simulink model "BuckBoost"  (R2018b)
settings: Solver=FixedStepDiscrete  StartTime=0.0  StopTime=10.0  RelTol=1e-3  EnableMultiTasking=on
libraries: HRTIMERS_Lib x12, GPIO_Lib x3, ADC_Lib x1, STM32_Config_Lib x1
settings Model: Creator=reynaudp  LastModifiedBy=fenard1
settings DataIOCC: LimitDataPoints=on  SaveFormat=Array
settings OptimizationCC: DefaultParameterBehavior=Inlined  LifeSpan=1
settings DebuggingCC: SolverPrmCheckMsg=warning  MultiTaskDSMMsg=none  AllowSymbolicDim=off  SFUnexpectedBacktrackingDiag=warning  SFNoUnconditionalDefaultTransitionDiag=warning  SFExecutionAtInitializationDiag=none
settings HardwareCC: ProdBitPerPointer=32  ProdBitPerSizeT=32  ProdBitPerPtrDiffT=32  ProdLargestAtomicInteger=Integer  ProdWordSize=32  ProdHWDeviceType=STMicroelectronics->STM32 32-bit Cortex-M
settings ModelReferenceCC: PropagateSignalLabelsOutOfModel=off
settings SFSimCC: SimUseLocalCustomCode=off  MATLABDynamicMemAlloc=off
settings RTWCC: SystemTargetFile=stm32.tlc  TemplateMakefile=stm32.tmf  Description=stm32 (Embedded Target)  GenerateReport=on  RTWUseLocalCustomCode=off
settings CodeAppCC: IgnoreCustomStorageClasses=off  CustomSymbolStrType=$N$R$M  SimulinkBlockComments=off
settings STFCustomTargetCC: CodeReplacementLibrary=ARM CMSIS SIN COS  ParMdlRefBuildCompliant=on  IncludeMdlTerminateFcn=off  CombineOutputUpdateFcns=on  ERTCustomFileBanners=on  SupportNonFinite=off  SupportComplex=off  SupportContinuousTime=off  SupportNonInlinedSFcns=off  RemoveResetFunc=on  MATLABClassNameForMDSCustomization=Simulink.SoftwareTarget.ERTCustomization  SystemTargetFile=stm32.tlc
settings ERTTargetCC: CodeReplacementLibrary=ARM CMSIS SIN COS  MultiwordLength=2048  CompOptLevelCompliant=off  ConcurrentExecutionCompliant=off  IncludeMdlTerminateFcn=off  SupportNonFinite=off  SupportComplex=off  ModelStepFunctionPrototypeControlCompliant=off  CPPClassGenCompliant=off  UseToolchainInfoCompliant=off  ERTSrcFileBannerTemplate=sourceFileTemplate.cgt  ERTHdrFileBannerTemplate=sourceFileTemplate.cgt  ERTDataSrcFileTemplate=sourceFileTemplate.cgt  ERTDataHdrFileTemplate=sourceFileTemplate.cgt  ERTCustomFileTemplate=customRoutineProcess.tlc  ConvertIfToSwitch=off  SuppressUnreachableDefaultCases=off
settings ConfigComp: CovMetricSettings=dw  CovHtmlReporting=on  CovSaveCumulativeToWorkspaceVar=on  CovSaveSingleToWorkspaceVar=on  CovExternalEMLEnable=off  CovSFcnEnable=off

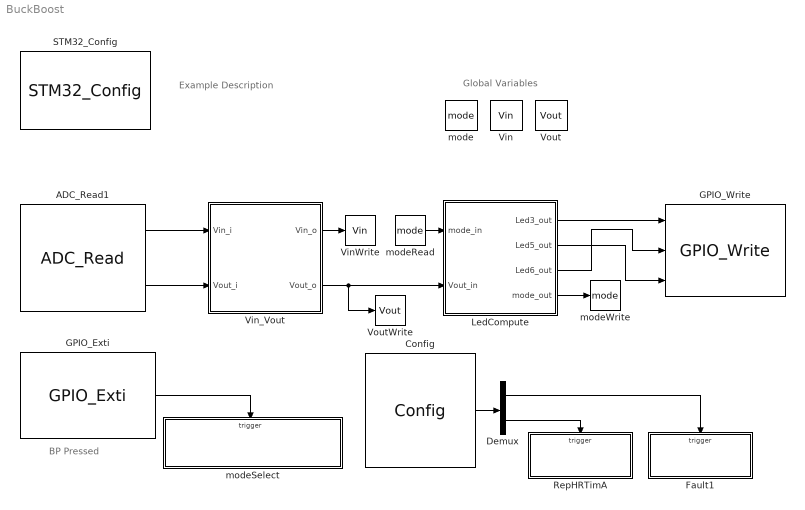
== system BuckBoost ==
  note: Example Description
  note: Global Variables
  note: BP Pressed
  ADC_Read1 : ADC_Lib/ADC_Read  ADC_Name=ADC1  ADC_Ch0=off  ADC_Ch1=off  ADC_Ch2=on  ADC_Ch3=off  ADC_Ch4=on  ADC_Ch5=off  ADC_Ch6=off  ADC_Ch7=off  ADC_Ch8=off  ADC_Ch9=off  ADC_Ch10=off  ADC_Ch11=off  ADC_Ch12=off  ADC_Ch13=off  ADC_Ch14=off  ADC_Ch15=off  ADC_Ch16=off  ADC_Ch17=off  ADC_Ch18=off  RgRk1=off  RgRk2=off  RgRk3=off  RgRk4=off  RgRk1_Ch=off  RgRk2_Ch=off  RgRk3_Ch=off  RgRk4_Ch=off  RgRk5=off  RgRk6=off  RgRk7=off  RgRk8=off  RgRk5_Ch=off  RgRk6_Ch=off  RgRk7_Ch=off  RgRk8_Ch=off  RgRk9=off  RgRk10=off  RgRk11=off  RgRk12=off  RgRk9_Ch=off  RgRk10_Ch=off  RgRk11_Ch=off  RgRk12_Ch=off  RgRk13=off  RgRk14=off  RgRk15=off  RgRk16=off  RgRk13_Ch=off  RgRk14_Ch=off  RgRk15_Ch=off  RgRk16_Ch=off  InjRk1=on  InjRk2=on  InjRk3=off  InjRk4=off  InjRk1_Ch=Ch2_i1  InjRk2_Ch=Ch4_i2  InjRk3_Ch=off  InjRk4_Ch=off  ADC_Trig=Not used  ADC_TrigEdge=Not used  DmaReq=off  DMA_Buffer=0  ItReq=off  AWD_Mode=NOT_USED  AWD_Ch=0  AWD_HThres=0  AWD_LThres=0  AWD_En_Int=off  AWD2_HThres=0  AWD2_LThres=0  AWD2_En_Int=off  AWD3_HThres=0  AWD3_LThres=0  AWD3_En_Int=off  EOC_SEQ=off  EOC_IT=off  JEOC_IT=off  AWD_IT=off  OVR_IT=off  CpltTrans=off  HalfTrans=off  ADC_RegNb=0  ADC_RegCh0=off  ADC_RegCh1=off  ADC_RegCh2=off  ADC_RegCh3=off  ADC_RegCh4=off  ADC_RegCh5=off  ADC_RegCh6=off  ADC_RegCh7=off  ADC_RegCh8=off  ADC_RegCh9=off  ADC_RegCh10=off  ADC_RegCh11=off  ADC_RegCh12=off  ADC_RegCh13=off  ADC_RegCh14=off  ADC_RegCh15=off  ADC_RegCh16=off  ADC_RegCh17=off  ADC_RegCh18=off  ADC_InjNb=2  ADC_InjCh0=off  ADC_InjCh1=off  ADC_InjCh2=on  ADC_InjCh3=off  ADC_InjCh4=on  ADC_InjCh5=off  ADC_InjCh6=off  ADC_InjCh7=off  ADC_InjCh8=off  ADC_InjCh9=off  ADC_InjCh10=off  ADC_InjCh11=off  ADC_InjCh12=off  ADC_InjCh13=off  ADC_InjCh14=off  ADC_InjCh15=off  ADC_InjCh16=off  ADC_InjCh17=off  ADC_InjCh18=off  ADC_RegRank0=0  ADC_RegRank1=0  ADC_RegRank2=0  ADC_RegRank3=0  ADC_RegRank4=0  ADC_RegRank5=0  ADC_RegRank6=0  ADC_RegRank7=0  ADC_RegRank8=0  ADC_RegRank9=0  ADC_RegRank10=0  ADC_RegRank11=0  ADC_RegRank12=0  ADC_RegRank13=0  ADC_RegRank14=0  ADC_RegRank15=0  ADC_RegRank16=0  ADC_RegRank17=0  ADC_RegRank18=0  ADC_InjRank0=0  ADC_InjRank1=0  ADC_InjRank2=1  ADC_InjRank3=0  ADC_InjRank4=2  ADC_InjRank5=0  ADC_InjRank6=0  ADC_InjRank7=0  ADC_InjRank8=0  ADC_InjRank9=0  ADC_InjRank10=0  ADC_InjRank11=0  ADC_InjRank12=0  ADC_InjRank13=0  ADC_InjRank14=0  ADC_InjRank15=0  ADC_InjRank16=0  ADC_InjRank17=0  ADC_InjRank18=0  NbADC=1  CurrentADC=ADC1
      settings: SourceProductName=Target Support Package - STM32 Adapter
  Config : HRTIMERS_Lib/Config  currentHRTIM=HRTIM1  NbHRTim=1  HRTIM_Name=HRTIM1  HRTIM_Clock=144000000  TIM_IRQ_F1=on  TIM_IRQ_F2=off  TIM_IRQ_F3=off  TIM_IRQ_F4=off  TIM_IRQ_F5=off  TIM_IRQ_F6=off  TIM_IRQ_SF=off  TIM_IRQ_BMP=off  TIM_IRQ_DLLCALL=off  TIM_IRQ_SYNC=off  TIM_IRQ_BURST_DMA=off  TIM_IRQ_DMA_ERR=off  M_DMA=off  M_IT_global=off  M_Tim_div=MUL32  M_Period=0  M_PWM_Period=Inf  M_Unit1=0  M_Unit2=0  M_Unit3=0  M_Unit4=0  TIM_IRQ_UPDM=off  TIM_IRQ_REPM=off  TIM_IRQ_COMP1=off  TIM_IRQ_COMP2=off  TIM_IRQ_COMP3=off  TIM_IRQ_COMP4=off  A_Mode=Advanced  A_DMA=off  A_IT_global=on  A_Tim_div=MUL32  A_Period=18432  A_PWM_Period=250000  A_Capture1=off  A_Capture2=off  TA1_Enable=on  TA1_Polarity=HIGH  TA1_Chopper=off  TA2_Enable=on  TA2_Polarity=HIGH  TA2_Chopper=off  A_Unit1=18336  A_Unit2=9216  A_Unit3=0  A_Unit4=0  A_Output_Comp1=off  A_Comp_Polarity1=HIGH  A_CompVal1=0  A_Output_Comp2=off  A_Comp_Polarity2=HIGH  A_CompVal2=0  A_Output_PWM1=off  A_Output_Polarity1=HIGH  A_DutyVal1=0  A_DutyIn1=off  A_Output_PWM2=off  A_Output_Polarity2=HIGH  A_DutyVal2=0  A_DutyIn2=off  A_OnePulse1=off  A_OnePulse_Polarity1=HIGH  A_OnePulse_CompVal1=0  A_OnePulse2=off  A_OnePulse_Polarity2=HIGH  A_OnePulse_CompVal2=0  TIM_IRQ_UPDA=off  TIM_IRQ_REPA=on  TIM_IRQ_COMP1A=off  TIM_IRQ_COMP2A=off  TIM_IRQ_COMP3A=off  TIM_IRQ_COMP4A=off  TIM_IRQ_CAPT1A=off  TIM_IRQ_CAPT2A=off  TIM_IRQ_DELA=off  TIM_IRQ_RESET_CPTA=off  TIM_IRQ_OUT1SA=off  TIM_IRQ_OUT1RA=off  TIM_IRQ_OUT2SA=off  TIM_IRQ_OUT2RA=off  B_Mode=Advanced  B_DMA=off  B_IT_global=off  B_Tim_div=MUL32  B_Period=18432  B_PWM_Period=250000  B_Capture1=off  B_Capture2=off  TB1_Enable=on  TB1_Polarity=HIGH  TB1_Chopper=off  TB2_Enable=on  TB2_Polarity=HIGH  TB2_Chopper=off  B_Unit1=18433  B_Unit2=0  B_Unit3=0  B_Unit4=0  B_Output_Comp1=off  B_Comp_Polarity1=HIGH  B_CompVal1=0  B_Output_Comp2=off  B_Comp_Polarity2=HIGH  B_CompVal2=0  B_Output_PWM1=off  B_Output_Polarity1=HIGH  B_DutyVal1=0  B_DutyIn1=off  B_Output_PWM2=off  B_Output_Polarity2=HIGH  B_DutyVal2=0  B_DutyIn2=off  B_OnePulse1=off  B_OnePulse_Polarity1=HIGH  B_OnePulse_CompVal1=0  B_OnePulse2=off  B_OnePulse_Polarity2=HIGH  B_OnePulse_CompVal2=0  TIM_IRQ_UPDB=off  TIM_IRQ_REPB=off  TIM_IRQ_COMP1B=off  TIM_IRQ_COMP2B=off  TIM_IRQ_COMP3B=off  TIM_IRQ_COMP4B=off  TIM_IRQ_CAPT1B=off  TIM_IRQ_CAPT2B=off  TIM_IRQ_DELB=off  TIM_IRQ_RESET_CPTB=off  TIM_IRQ_OUT1SB=off  TIM_IRQ_OUT1RB=off  TIM_IRQ_OUT2SB=off  TIM_IRQ_OUT2RB=off  C_Mode=Advanced  C_DMA=off  C_IT_global=off  C_Tim_div=MUL32  C_Period=0  C_PWM_Period=Inf  C_Capture1=off  C_Capture2=off  TC1_Enable=off  TC1_Polarity=HIGH  TC1_Chopper=off  TC2_Enable=off  TC2_Polarity=HIGH  TC2_Chopper=off  C_Unit1=0  C_Unit2=0  C_Unit3=0  C_Unit4=0  C_Output_Comp1=off  C_Comp_Polarity1=HIGH  C_CompVal1=0  C_Output_Comp2=off  C_Comp_Polarity2=HIGH  C_CompVal2=0  C_Output_PWM1=off  C_Output_Polarity1=HIGH  C_DutyVal1=0  C_DutyIn1=off  C_Output_PWM2=off  C_Output_Polarity2=HIGH  C_DutyVal2=0  C_DutyIn2=off  C_OnePulse1=off  C_OnePulse_Polarity1=HIGH  C_OnePulse_CompVal1=0  C_OnePulse2=off  C_OnePulse_Polarity2=HIGH  C_OnePulse_CompVal2=0  TIM_IRQ_UPDC=off  TIM_IRQ_REPC=off  TIM_IRQ_COMP1C=off  TIM_IRQ_COMP2C=off  TIM_IRQ_COMP3C=off  TIM_IRQ_COMP4C=off  TIM_IRQ_CAPT1C=off  TIM_IRQ_CAPT2C=off  TIM_IRQ_DELC=off  TIM_IRQ_RESET_CPTC=off  TIM_IRQ_OUT1SC=off  TIM_IRQ_OUT1RC=off  TIM_IRQ_OUT2SC=off  TIM_IRQ_OUT2RC=off  D_Mode=Advanced  D_DMA=off  D_IT_global=off  D_Tim_div=MUL32  D_Period=0  D_PWM_Period=Inf  D_Capture1=off  D_Capture2=off  TD1_Enable=off  TD1_Polarity=HIGH  TD1_Chopper=off  TD2_Enable=off  TD2_Polarity=HIGH  TD2_Chopper=off  D_Unit1=0  D_Unit2=0  D_Unit3=0  D_Unit4=0  D_Output_Comp1=off  D_Comp_Polarity1=HIGH  D_CompVal1=0  D_Output_Comp2=off  D_Comp_Polarity2=HIGH  D_CompVal2=0  D_Output_PWM1=off  D_Output_Polarity1=HIGH  D_DutyVal1=0  D_DutyIn1=off  D_Output_PWM2=off  D_Output_Polarity2=HIGH  D_DutyVal2=0  D_DutyIn2=off  D_OnePulse1=off  D_OnePulse_Polarity1=HIGH  D_OnePulse_CompVal1=0  D_OnePulse2=off  D_OnePulse_Polarity2=HIGH  D_OnePulse_CompVal2=0  TIM_IRQ_UPDD=off  TIM_IRQ_REPD=off  TIM_IRQ_COMP1D=off  TIM_IRQ_COMP2D=off  TIM_IRQ_COMP3D=off  TIM_IRQ_COMP4D=off  TIM_IRQ_CAPT1D=off  TIM_IRQ_CAPT2D=off  TIM_IRQ_DELD=off  TIM_IRQ_RESET_CPTD=off  TIM_IRQ_OUT1SD=off  TIM_IRQ_OUT1RD=off  TIM_IRQ_OUT2SD=off  TIM_IRQ_OUT2RD=off  E_Mode=Advanced  E_DMA=off  E_IT_global=off  E_Tim_div=MUL32  E_Period=0  E_PWM_Period=Inf  E_Capture1=off  E_Capture2=off  TE1_Enable=off  TE1_Polarity=HIGH  TE1_Chopper=off  TE2_Enable=off  TE2_Polarity=HIGH  TE2_Chopper=off  E_Unit1=0  E_Unit2=0  E_Unit3=0  E_Unit4=0  E_Output_Comp1=off  E_Comp_Polarity1=HIGH  E_CompVal1=0  E_Output_Comp2=off  E_Comp_Polarity2=HIGH  E_CompVal2=0  E_Output_PWM1=off  E_Output_Polarity1=HIGH  E_DutyVal1=0  E_DutyIn1=off  E_Output_PWM2=off  E_Output_Polarity2=HIGH  E_DutyVal2=0  E_DutyIn2=off  E_OnePulse1=off  E_OnePulse_Polarity1=HIGH  E_OnePulse_CompVal1=0  E_OnePulse2=off  E_OnePulse_Polarity2=HIGH  E_OnePulse_CompVal2=0  TIM_IRQ_UPDE=off  TIM_IRQ_REPE=off  TIM_IRQ_COMP1E=off  TIM_IRQ_COMP2E=off  TIM_IRQ_COMP3E=off  TIM_IRQ_COMP4E=off  TIM_IRQ_CAPT1E=off  TIM_IRQ_CAPT2E=off  TIM_IRQ_DELE=off  TIM_IRQ_RESET_CPTE=off  TIM_IRQ_OUT1SE=off  TIM_IRQ_OUT1RE=off  TIM_IRQ_OUT2SE=off  TIM_IRQ_OUT2RE=off  F_Mode=Advanced  F_DMA=off  F_IT_global=off  F_Tim_div=MUL32  F_Period=0  F_PWM_Period=Inf  F_Capture1=off  F_Capture2=off  TF1_Enable=off  TF1_Polarity=HIGH  TF1_Chopper=off  TF2_Enable=off  TF2_Polarity=HIGH  TF2_Chopper=off  F_Unit1=0  F_Unit2=0  F_Unit3=0  F_Unit4=0  F_Output_Comp1=off  F_Comp_Polarity1=HIGH  F_CompVal1=0  F_Output_Comp2=off  F_Comp_Polarity2=HIGH  F_CompVal2=0  F_Output_PWM1=off  F_Output_Polarity1=HIGH  F_DutyVal1=0  F_DutyIn1=off  F_Output_PWM2=off  F_Output_Polarity2=HIGH  F_DutyVal2=0  F_DutyIn2=off  F_OnePulse1=off  F_OnePulse_Polarity1=HIGH  F_OnePulse_CompVal1=0  F_OnePulse2=off  F_OnePulse_Polarity2=HIGH  F_OnePulse_CompVal2=0  TIM_IRQ_UPDF=off  TIM_IRQ_REPF=off  TIM_IRQ_COMP1F=off  TIM_IRQ_COMP2F=off  TIM_IRQ_COMP3F=off  TIM_IRQ_COMP4F=off  TIM_IRQ_CAPT1F=off  TIM_IRQ_CAPT2F=off  TIM_IRQ_DELF=off  TIM_IRQ_RESET_CPTF=off  TIM_IRQ_OUT1SF=off  TIM_IRQ_OUT1RF=off  TIM_IRQ_OUT2SF=off  TIM_IRQ_OUT2RF=off  M_Used=off  A_Used=on  B_Used=on  C_Used=off  D_Used=off  E_Used=off  F_Used=off
      settings: SourceProductName=Target Support Package - STM32 Adapter
  Demux : Demux  Outputs=2
  Fault1 : Subsystem  TreatAsAtomicUnit=on
  GPIO_Exti : GPIO_Lib/GPIO_Exti  Priority=0  Port_name=GPIOA  Pin_0=on  Pin_1=off  Pin_2=off  Pin_3=off  Pin_4=off  Pin_5=off  Pin_6=off  Pin_7=off  Pin_8=off  Pin_9=off  Pin_10=off  Pin_11=off  Pin_12=off  Pin_13=off  Pin_14=off  Pin_15=off  PinList=GPIOA0
      settings: SourceProductName=Target Support Package - STM32 Adapter
  GPIO_Write : GPIO_Lib/GPIO_Write  Port_name=GPIOB  Pin0=off  Toggle_Pin0=off  Pin1=off  Toggle_Pin1=off  Pin2=off  Toggle_Pin2=off  Pin3=off  Toggle_Pin3=off  Pin4=off  Toggle_Pin4=off  Pin5=off  Toggle_Pin5=off  Pin6=on  Toggle_Pin6=off  Pin7=on  Toggle_Pin7=off  Pin8=off  Toggle_Pin8=off  Pin9=on  Toggle_Pin9=off  Pin10=off  Toggle_Pin10=off  Pin11=off  Toggle_Pin11=off  Pin12=off  Toggle_Pin12=off  Pin13=off  Toggle_Pin13=off  Pin14=off  Toggle_Pin14=off  Pin15=off  Toggle_Pin15=off  PinList="GPIOB6  7  8  9"
      settings: SourceProductName=Target Support Package - STM32 Adapter
  LedCompute : MATLAB Function  TreatAsAtomicUnit=on
  RepHRTimA : Subsystem  TreatAsAtomicUnit=on
  STM32_Config : STM32_Config_Lib/STM32_Config  Priority=0  Project_Path=.\  Config_File=BuckBoost.ioc  MCU_Name=STM32F334C8Tx
      settings: SourceProductName=Target Support Package - STM32 Adapter
  Vin : DataStoreMemory  DataStoreName=Vin  ReadBeforeWriteMsg=warning  WriteAfterWriteMsg=warning  WriteAfterReadMsg=warning  ShowAdditionalParam=off  OutMin=0  OutMax=5000  OutDataTypeStr=uint32
  VinWrite : DataStoreWrite  DataStoreName=Vin
  Vin_Vout : MATLAB Function  TreatAsAtomicUnit=on
  Vout : DataStoreMemory  DataStoreName=Vout  ReadBeforeWriteMsg=warning  WriteAfterWriteMsg=warning  WriteAfterReadMsg=warning  ShowAdditionalParam=off  OutMin=0  OutDataTypeStr=uint32
  VoutWrite : DataStoreWrite  DataStoreName=Vout
  mode : DataStoreMemory  DataStoreName=mode  ReadBeforeWriteMsg=warning  WriteAfterWriteMsg=warning  WriteAfterReadMsg=warning  ShowAdditionalParam=off  OutMin=0  OutMax=3  OutDataTypeStr=uint8
  modeRead : DataStoreRead  DataStoreName=mode
  modeSelect : Subsystem  TreatAsAtomicUnit=on
  modeWrite : DataStoreWrite  DataStoreName=mode
  wires:
  GPIO_Exti/1 -> modeSelect/Trigger
  ADC_Read1/2 -> Vin_Vout/2(Vout_i)
  ADC_Read1/1 -> Vin_Vout/1(Vin_i)
  Vin_Vout/1(Vin_o) -> VinWrite/1
  Vin_Vout/2(Vout_o) -> VoutWrite/1, LedCompute/2(Vout_in)
  modeRead/1 -> LedCompute/1(mode_in)
  LedCompute/4(mode_out) -> modeWrite/1
  LedCompute/1(Led3_out) -> GPIO_Write/1
  LedCompute/2(Led5_out) -> GPIO_Write/3
  LedCompute/3(Led6_out) -> GPIO_Write/2
  Config/1 -> Demux/1
  Demux/1 -> Fault1/Trigger
  Demux/2 -> RepHRTimA/Trigger

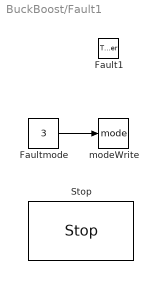
== system BuckBoost/Fault1 ==
  Fault1 : TriggerPort  TriggerType=function-call  VariantControl=Variant
  Faultmode : Constant  Value=3  OutDataTypeStr=uint8
  Stop : HRTIMERS_Lib/Stop  currentHRTIM=HRTIM1  NbHRTim=1  HRTIM_Name=HRTIM1  TA1_Stop=on  TA2_Stop=on  TB1_Stop=on  TB2_Stop=on  TC1_Stop=off  TC2_Stop=off  TD1_Stop=off  TD2_Stop=off  TE1_Stop=off  TE2_Stop=off  TF1_Stop=off  TF2_Stop=off
      settings: SourceProductName=Target Support Package - STM32 Adapter
  modeWrite : DataStoreWrite  DataStoreName=mode
  wires:
  Faultmode/1 -> modeWrite/1

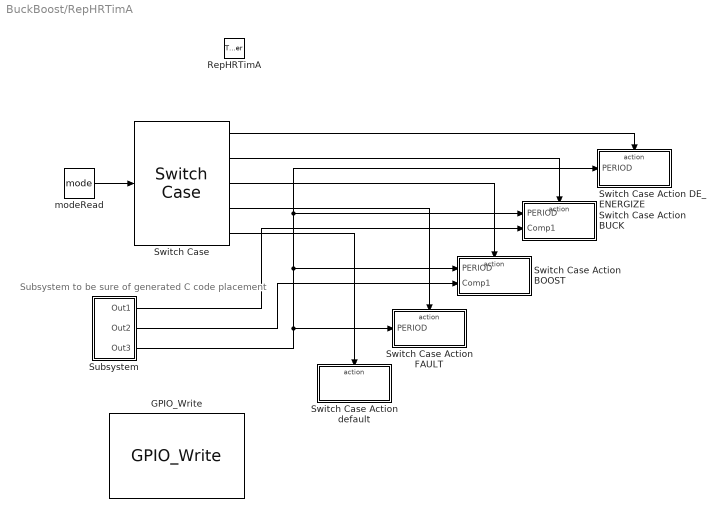
== system BuckBoost/RepHRTimA ==
  note: Subsystem to be sure of generated C code placement
  RepHRTimA : TriggerPort  TriggerType=function-call  VariantControl=Variant
  GPIO_Write : GPIO_Lib/GPIO_Write  Port_name=GPIOB  Pin0=off  Toggle_Pin0=off  Pin1=off  Toggle_Pin1=off  Pin2=off  Toggle_Pin2=off  Pin3=off  Toggle_Pin3=off  Pin4=off  Toggle_Pin4=off  Pin5=off  Toggle_Pin5=off  Pin6=off  Toggle_Pin6=off  Pin7=off  Toggle_Pin7=off  Pin8=on  Toggle_Pin8=on  Pin9=off  Toggle_Pin9=off  Pin10=off  Toggle_Pin10=off  Pin11=off  Toggle_Pin11=off  Pin12=off  Toggle_Pin12=off  Pin13=off  Toggle_Pin13=off  Pin14=off  Toggle_Pin14=off  Pin15=off  Toggle_Pin15=off  PinList="GPIOB6  7  8  9"
      settings: SourceProductName=Target Support Package - STM32 Adapter
  Subsystem : Subsystem  TreatAsAtomicUnit=on
      settings: RTWSystemCode=Inline
  Switch Case : SwitchCase  Priority=0  CaseConditions={0,1,2,3}
  Switch Case Action BOOST : Subsystem  TreatAsAtomicUnit=on
  Switch Case Action BUCK : Subsystem  TreatAsAtomicUnit=on
  Switch Case Action DE_ENERGIZE : Subsystem  TreatAsAtomicUnit=on
  Switch Case Action FAULT : Subsystem  TreatAsAtomicUnit=on
  Switch Case Action default : Subsystem  TreatAsAtomicUnit=on
  modeRead : DataStoreRead  DataStoreName=mode
  wires:
  modeRead/1 -> Switch Case/1
  Switch Case/2 -> Switch Case Action BUCK/Action
  Switch Case/3 -> Switch Case Action BOOST/Action
  Switch Case/4 -> Switch Case Action FAULT/Action
  Switch Case/1 -> Switch Case Action DE_ENERGIZE/Action
  Switch Case/5 -> Switch Case Action default/Action
  Subsystem/3(Out3) -> Switch Case Action BOOST/1(PERIOD), Switch Case Action BUCK/1(PERIOD), Switch Case Action DE_ENERGIZE/1(PERIOD), Switch Case Action FAULT/1(PERIOD)
  Subsystem/1(Out1) -> Switch Case Action BUCK/2(Comp1)
  Subsystem/2(Out2) -> Switch Case Action BOOST/2(Comp1)

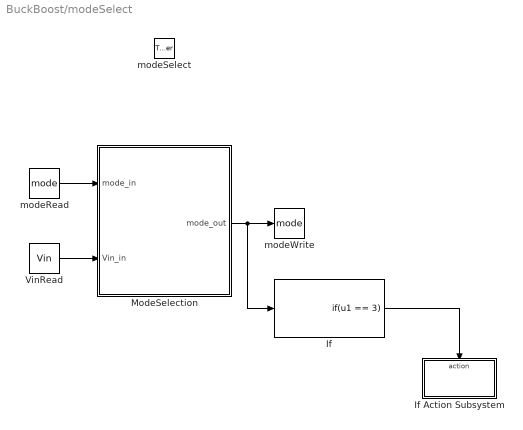
== system BuckBoost/modeSelect ==
  modeSelect : TriggerPort  TriggerType=function-call  VariantControl=Variant
  If : If  IfExpression=u1 == 3  ShowElse=off
  If Action Subsystem : Subsystem  TreatAsAtomicUnit=on
  ModeSelection : MATLAB Function  TreatAsAtomicUnit=on
  VinRead : DataStoreRead  DataStoreName=Vin
  modeRead : DataStoreRead  DialogController=Simulink.DDGSource  DataStoreName=mode
  modeWrite : DataStoreWrite  DataStoreName=mode
  wires:
  modeRead/1 -> ModeSelection/1(mode_in)
  VinRead/1 -> ModeSelection/2(Vin_in)
  ModeSelection/1(mode_out) -> If/1, modeWrite/1
  If/1 -> If Action Subsystem/Action

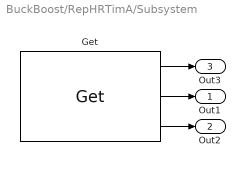
== system BuckBoost/RepHRTimA/Subsystem ==
  Get : HRTIMERS_Lib/Get  Priority=-1  currentHRTIM=HRTIM1  NbHRTim=1  HRTIM_Name=HRTIM1  M_Used=off  M_Period=off  M_Comp1=off  M_Comp2=off  M_Comp3=off  M_Comp4=off  A_Used=on  A_Period=on  A_Capt1_In=off  A_Capt2_In=off  A_Info=Timer A TA1 and TA2 lines are not configured as input.  A_Comp1=on  A_Comp2=off  A_Comp3=off  A_Comp4=off  B_Used=on  B_Period=off  B_Capt1_In=off  B_Capt2_In=off  B_Info=Timer B TB1 and TB2 lines are not configured as input.  B_Comp1=on  B_Comp2=off  B_Comp3=off  B_Comp4=off  C_Used=off  C_Period=off  C_Capt1_In=off  C_Capt2_In=off  C_Info=Timer C is not configured.  C_Comp1=off  C_Comp2=off  C_Comp3=off  C_Comp4=off  D_Used=off  D_Period=off  D_Capt1_In=off  D_Capt2_In=off  D_Info=Timer D is not configured.  D_Comp1=off  D_Comp2=off  D_Comp3=off  D_Comp4=off  E_Used=off  E_Period=off  E_Capt1_In=off  E_Capt2_In=off  E_Info=Timer E is not configured.  E_Comp1=off  E_Comp2=off  E_Comp3=off  E_Comp4=off  F_Used=off  F_Period=off  F_Capt1_In=off  F_Capt2_In=off  F_Info=Timer F is not configured.  F_Comp1=off  F_Comp2=off  F_Comp3=off  F_Comp4=off
      settings: SourceProductName=Target Support Package - STM32 Adapter
  Out1 : Outport
  Out2 : Outport  Port=2
  Out3 : Outport  Port=3
  wires:
  Get/1 -> Out3/1
  Get/2 -> Out1/1
  Get/3 -> Out2/1

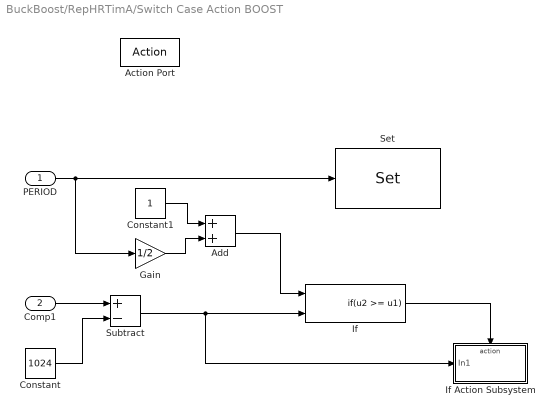
== system BuckBoost/RepHRTimA/Switch Case Action BOOST ==
  PERIOD : Inport
  Comp1 : Inport  Port=2
  Action Port : ActionPort  ActionType=case
  Add : Sum
  Constant : Constant  Value=1024
  Constant1 : Constant
  Gain : Gain  Gain=1/2
  If : If  NumInputs=2  IfExpression=u2 >= u1  ShowElse=off
  If Action Subsystem : Subsystem  TreatAsAtomicUnit=on
  Set : HRTIMERS_Lib/Set  currentHRTIM=HRTIM1  NbHRTim=1  HRTIM_Name=HRTIM1  M_Used=off  M_Comp1_In=off  M_Comp1=0  M_Comp2_In=off  M_Comp2=0  M_Comp3_In=off  M_Comp3=0  M_Comp4_In=off  M_Comp4=0  A_Used=on  A_Comp1_In=on  A_Comp1=0  A_Comp2_In=off  A_Comp2=0  A_Comp3_In=off  A_Comp3=0  A_Comp4_In=off  A_Comp4=0  B_Used=on  B_Comp1_In=off  B_Comp1=0  B_Comp2_In=off  B_Comp2=0  B_Comp3_In=off  B_Comp3=0  B_Comp4_In=off  B_Comp4=0  C_Used=off  C_Comp1_In=off  C_Comp1=0  C_Comp2_In=off  C_Comp2=0  C_Comp3_In=off  C_Comp3=0  C_Comp4_In=off  C_Comp4=0  D_Used=off  D_Comp1_In=off  D_Comp1=0  D_Comp2_In=off  D_Comp2=0  D_Comp3_In=off  D_Comp3=0  D_Comp4_In=off  D_Comp4=0  E_Used=off  E_Comp1_In=off  E_Comp1=0  E_Comp2_In=off  E_Comp2=0  E_Comp3_In=off  E_Comp3=0  E_Comp4_In=off  E_Comp4=0  F_Used=off  F_Comp1_In=off  F_Comp1=0  F_Comp2_In=off  F_Comp2=0  F_Comp3_In=off  F_Comp3=0  F_Comp4_In=off  F_Comp4=0
      settings: SourceProductName=Target Support Package - STM32 Adapter
  Subtract : Sum  Inputs=+-
  wires:
  PERIOD/1 -> Gain/1, Set/1
  Comp1/1 -> Subtract/1
  Constant/1 -> Subtract/2
  Constant1/1 -> Add/1
  Gain/1 -> Add/2
  Add/1 -> If/1
  Subtract/1 -> If Action Subsystem/1(In1), If/2
  If/1 -> If Action Subsystem/Action

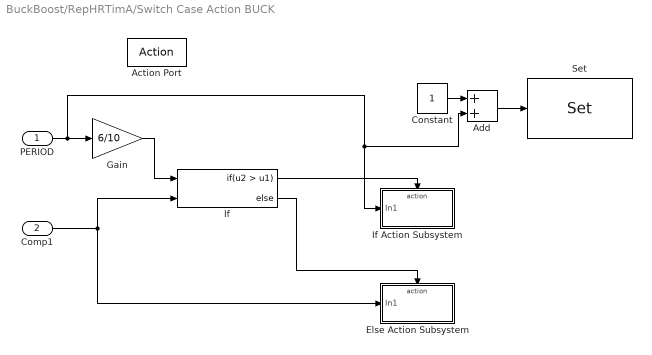
== system BuckBoost/RepHRTimA/Switch Case Action BUCK ==
  PERIOD : Inport
  Comp1 : Inport  Port=2
  Action Port : ActionPort  ActionType=case
  Add : Sum
  Constant : Constant
  Else Action Subsystem : Subsystem  TreatAsAtomicUnit=on
  Gain : Gain  Gain=6/10
  If : If  NumInputs=2  IfExpression=u2 > u1
  "If Action Subsystem " : Subsystem  TreatAsAtomicUnit=on
  Set : HRTIMERS_Lib/Set  currentHRTIM=HRTIM1  NbHRTim=1  HRTIM_Name=HRTIM1  M_Used=off  M_Comp1_In=off  M_Comp1=0  M_Comp2_In=off  M_Comp2=0  M_Comp3_In=off  M_Comp3=0  M_Comp4_In=off  M_Comp4=0  A_Used=on  A_Comp1_In=off  A_Comp1=0  A_Comp2_In=off  A_Comp2=0  A_Comp3_In=off  A_Comp3=0  A_Comp4_In=off  A_Comp4=0  B_Used=on  B_Comp1_In=on  B_Comp1=0  B_Comp2_In=off  B_Comp2=0  B_Comp3_In=off  B_Comp3=0  B_Comp4_In=off  B_Comp4=0  C_Used=off  C_Comp1_In=off  C_Comp1=0  C_Comp2_In=off  C_Comp2=0  C_Comp3_In=off  C_Comp3=0  C_Comp4_In=off  C_Comp4=0  D_Used=off  D_Comp1_In=off  D_Comp1=0  D_Comp2_In=off  D_Comp2=0  D_Comp3_In=off  D_Comp3=0  D_Comp4_In=off  D_Comp4=0  E_Used=off  E_Comp1_In=off  E_Comp1=0  E_Comp2_In=off  E_Comp2=0  E_Comp3_In=off  E_Comp3=0  E_Comp4_In=off  E_Comp4=0  F_Used=off  F_Comp1_In=off  F_Comp1=0  F_Comp2_In=off  F_Comp2=0  F_Comp3_In=off  F_Comp3=0  F_Comp4_In=off  F_Comp4=0
      settings: SourceProductName=Target Support Package - STM32 Adapter
  wires:
  Comp1/1 -> Else Action Subsystem/1(In1), If/2
  PERIOD/1 -> "If Action Subsystem "/1(In1), Add/2, Gain/1
  Gain/1 -> If/1
  If/1 -> "If Action Subsystem "/Action
  If/2 -> Else Action Subsystem/Action
  Add/1 -> Set/1
  Constant/1 -> Add/1

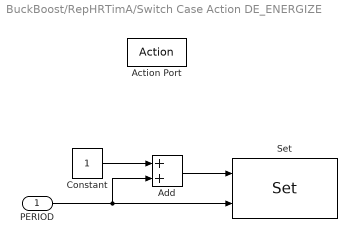
== system BuckBoost/RepHRTimA/Switch Case Action DE_ENERGIZE ==
  PERIOD : Inport
  Action Port : ActionPort  ActionType=case
  Add : Sum
  Constant : Constant
  Set : HRTIMERS_Lib/Set  currentHRTIM=HRTIM1  NbHRTim=1  HRTIM_Name=HRTIM1  M_Used=off  M_Comp1_In=off  M_Comp1=0  M_Comp2_In=off  M_Comp2=0  M_Comp3_In=off  M_Comp3=0  M_Comp4_In=off  M_Comp4=0  A_Used=on  A_Comp1_In=on  A_Comp1=0  A_Comp2_In=off  A_Comp2=0  A_Comp3_In=off  A_Comp3=0  A_Comp4_In=off  A_Comp4=0  B_Used=on  B_Comp1_In=on  B_Comp1=0  B_Comp2_In=off  B_Comp2=0  B_Comp3_In=off  B_Comp3=0  B_Comp4_In=off  B_Comp4=0  C_Used=off  C_Comp1_In=off  C_Comp1=0  C_Comp2_In=off  C_Comp2=0  C_Comp3_In=off  C_Comp3=0  C_Comp4_In=off  C_Comp4=0  D_Used=off  D_Comp1_In=off  D_Comp1=0  D_Comp2_In=off  D_Comp2=0  D_Comp3_In=off  D_Comp3=0  D_Comp4_In=off  D_Comp4=0  E_Used=off  E_Comp1_In=off  E_Comp1=0  E_Comp2_In=off  E_Comp2=0  E_Comp3_In=off  E_Comp3=0  E_Comp4_In=off  E_Comp4=0  F_Used=off  F_Comp1_In=off  F_Comp1=0  F_Comp2_In=off  F_Comp2=0  F_Comp3_In=off  F_Comp3=0  F_Comp4_In=off  F_Comp4=0
      settings: SourceProductName=Target Support Package - STM32 Adapter
  wires:
  PERIOD/1 -> Add/2, Set/2
  Add/1 -> Set/1
  Constant/1 -> Add/1

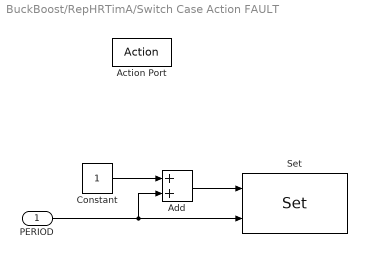
== system BuckBoost/RepHRTimA/Switch Case Action FAULT ==
  PERIOD : Inport
  Action Port : ActionPort  ActionType=case
  Add : Sum
  Constant : Constant
  Set : HRTIMERS_Lib/Set  currentHRTIM=HRTIM1  NbHRTim=1  HRTIM_Name=HRTIM1  M_Used=off  M_Comp1_In=off  M_Comp1=0  M_Comp2_In=off  M_Comp2=0  M_Comp3_In=off  M_Comp3=0  M_Comp4_In=off  M_Comp4=0  A_Used=on  A_Comp1_In=on  A_Comp1=0  A_Comp2_In=off  A_Comp2=0  A_Comp3_In=off  A_Comp3=0  A_Comp4_In=off  A_Comp4=0  B_Used=on  B_Comp1_In=on  B_Comp1=0  B_Comp2_In=off  B_Comp2=0  B_Comp3_In=off  B_Comp3=0  B_Comp4_In=off  B_Comp4=0  C_Used=off  C_Comp1_In=off  C_Comp1=0  C_Comp2_In=off  C_Comp2=0  C_Comp3_In=off  C_Comp3=0  C_Comp4_In=off  C_Comp4=0  D_Used=off  D_Comp1_In=off  D_Comp1=0  D_Comp2_In=off  D_Comp2=0  D_Comp3_In=off  D_Comp3=0  D_Comp4_In=off  D_Comp4=0  E_Used=off  E_Comp1_In=off  E_Comp1=0  E_Comp2_In=off  E_Comp2=0  E_Comp3_In=off  E_Comp3=0  E_Comp4_In=off  E_Comp4=0  F_Used=off  F_Comp1_In=off  F_Comp1=0  F_Comp2_In=off  F_Comp2=0  F_Comp3_In=off  F_Comp3=0  F_Comp4_In=off  F_Comp4=0
      settings: SourceProductName=Target Support Package - STM32 Adapter
  wires:
  Add/1 -> Set/1
  Constant/1 -> Add/1
  PERIOD/1 -> Set/2, Add/2

== system BuckBoost/RepHRTimA/Switch Case Action default ==
  Action Port : ActionPort  ActionType=default
  Disable : HRTIMERS_Lib/Disable  currentHRTIM=HRTIM1  NbHRTim=1  HRTIM_Name=HRTIM1  M_Disable=off  A_Disable=on  B_Disable=on  C_Disable=off  D_Disable=off  E_Disable=off  F_Disable=off
      settings: SourceProductName=Target Support Package - STM32 Adapter

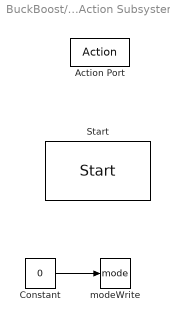
== system BuckBoost/modeSelect/If Action Subsystem ==
  Action Port : ActionPort  ActionType=then
  Constant : Constant  Value=0  OutDataTypeStr=uint8
  Start : HRTIMERS_Lib/Start  currentHRTIM=HRTIM1  NbHRTim=1  HRTIM_Name=HRTIM1  TA1_Start=on  TA2_Start=on  TB1_Start=on  TB2_Start=on  TC1_Start=off  TC2_Start=off  TD1_Start=off  TD2_Start=off  TE1_Start=off  TE2_Start=off  TF1_Start=off  TF2_Start=off
      settings: SourceProductName=Target Support Package - STM32 Adapter
  modeWrite : DataStoreWrite  DataStoreName=mode
  wires:
  Constant/1 -> modeWrite/1

== system BuckBoost/RepHRTimA/Switch Case Action BOOST/If Action Subsystem ==
  In1 : Inport
  Action Port : ActionPort  ActionType=then
  Set : HRTIMERS_Lib/Set  currentHRTIM=HRTIM1  NbHRTim=1  HRTIM_Name=HRTIM1  M_Used=off  M_Comp1_In=off  M_Comp1=0  M_Comp2_In=off  M_Comp2=0  M_Comp3_In=off  M_Comp3=0  M_Comp4_In=off  M_Comp4=0  A_Used=on  A_Comp1_In=off  A_Comp1=0  A_Comp2_In=off  A_Comp2=0  A_Comp3_In=off  A_Comp3=0  A_Comp4_In=off  A_Comp4=0  B_Used=on  B_Comp1_In=on  B_Comp1=0  B_Comp2_In=off  B_Comp2=0  B_Comp3_In=off  B_Comp3=0  B_Comp4_In=off  B_Comp4=0  C_Used=off  C_Comp1_In=off  C_Comp1=0  C_Comp2_In=off  C_Comp2=0  C_Comp3_In=off  C_Comp3=0  C_Comp4_In=off  C_Comp4=0  D_Used=off  D_Comp1_In=off  D_Comp1=0  D_Comp2_In=off  D_Comp2=0  D_Comp3_In=off  D_Comp3=0  D_Comp4_In=off  D_Comp4=0  E_Used=off  E_Comp1_In=off  E_Comp1=0  E_Comp2_In=off  E_Comp2=0  E_Comp3_In=off  E_Comp3=0  E_Comp4_In=off  E_Comp4=0  F_Used=off  F_Comp1_In=off  F_Comp1=0  F_Comp2_In=off  F_Comp2=0  F_Comp3_In=off  F_Comp3=0  F_Comp4_In=off  F_Comp4=0
      settings: SourceProductName=Target Support Package - STM32 Adapter
  wires:
  In1/1 -> Set/1

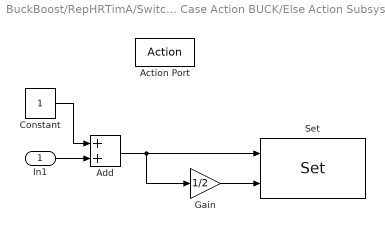
== system BuckBoost/RepHRTimA/Switch Case Action BUCK/Else Action Subsystem ==
  In1 : Inport
  Action Port : ActionPort  ActionType=else
  Add : Sum
  Constant : Constant
  Gain : Gain  Gain=1/2
  Set : HRTIMERS_Lib/Set  currentHRTIM=HRTIM1  NbHRTim=1  HRTIM_Name=HRTIM1  M_Used=off  M_Comp1_In=off  M_Comp1=0  M_Comp2_In=off  M_Comp2=0  M_Comp3_In=off  M_Comp3=0  M_Comp4_In=off  M_Comp4=0  A_Used=on  A_Comp1_In=on  A_Comp1=0  A_Comp2_In=on  A_Comp2=0  A_Comp3_In=off  A_Comp3=0  A_Comp4_In=off  A_Comp4=0  B_Used=on  B_Comp1_In=off  B_Comp1=0  B_Comp2_In=off  B_Comp2=0  B_Comp3_In=off  B_Comp3=0  B_Comp4_In=off  B_Comp4=0  C_Used=off  C_Comp1_In=off  C_Comp1=0  C_Comp2_In=off  C_Comp2=0  C_Comp3_In=off  C_Comp3=0  C_Comp4_In=off  C_Comp4=0  D_Used=off  D_Comp1_In=off  D_Comp1=0  D_Comp2_In=off  D_Comp2=0  D_Comp3_In=off  D_Comp3=0  D_Comp4_In=off  D_Comp4=0  E_Used=off  E_Comp1_In=off  E_Comp1=0  E_Comp2_In=off  E_Comp2=0  E_Comp3_In=off  E_Comp3=0  E_Comp4_In=off  E_Comp4=0  F_Used=off  F_Comp1_In=off  F_Comp1=0  F_Comp2_In=off  F_Comp2=0  F_Comp3_In=off  F_Comp3=0  F_Comp4_In=off  F_Comp4=0
      settings: SourceProductName=Target Support Package - STM32 Adapter
  wires:
  In1/1 -> Add/2
  Constant/1 -> Add/1
  Add/1 -> Gain/1, Set/1
  Gain/1 -> Set/2

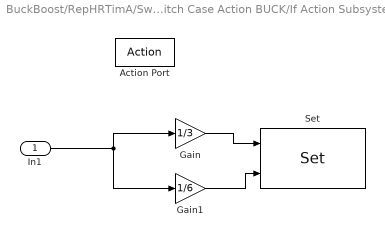
== system BuckBoost/RepHRTimA/Switch Case Action BUCK/If Action Subsystem  ==
  In1 : Inport
  Action Port : ActionPort  ActionType=then
  Gain : Gain  Gain=1/3
  Gain1 : Gain  Gain=1/6
  Set : HRTIMERS_Lib/Set  currentHRTIM=HRTIM1  NbHRTim=1  HRTIM_Name=HRTIM1  M_Used=off  M_Comp1_In=off  M_Comp1=0  M_Comp2_In=off  M_Comp2=0  M_Comp3_In=off  M_Comp3=0  M_Comp4_In=off  M_Comp4=0  A_Used=on  A_Comp1_In=on  A_Comp1=0  A_Comp2_In=on  A_Comp2=0  A_Comp3_In=off  A_Comp3=0  A_Comp4_In=off  A_Comp4=0  B_Used=on  B_Comp1_In=off  B_Comp1=0  B_Comp2_In=off  B_Comp2=0  B_Comp3_In=off  B_Comp3=0  B_Comp4_In=off  B_Comp4=0  C_Used=off  C_Comp1_In=off  C_Comp1=0  C_Comp2_In=off  C_Comp2=0  C_Comp3_In=off  C_Comp3=0  C_Comp4_In=off  C_Comp4=0  D_Used=off  D_Comp1_In=off  D_Comp1=0  D_Comp2_In=off  D_Comp2=0  D_Comp3_In=off  D_Comp3=0  D_Comp4_In=off  D_Comp4=0  E_Used=off  E_Comp1_In=off  E_Comp1=0  E_Comp2_In=off  E_Comp2=0  E_Comp3_In=off  E_Comp3=0  E_Comp4_In=off  E_Comp4=0  F_Used=off  F_Comp1_In=off  F_Comp1=0  F_Comp2_In=off  F_Comp2=0  F_Comp3_In=off  F_Comp3=0  F_Comp4_In=off  F_Comp4=0
      settings: SourceProductName=Target Support Package - STM32 Adapter
  wires:
  Gain/1 -> Set/1
  Gain1/1 -> Set/2
  In1/1 -> Gain/1, Gain1/1

== matlab function BuckBoost/modeSelect/ModeSelection ==
  data: mode_in input uint8; mode_out output uint8; Vin_in input uint32
function mode_out = ModeSelection(mode_in, Vin_in)
%#codegen
mode_out = mode_in;
switch mode_in
    case 0 
        %DE_ENERGISE mode
        mode_out = uint8(0);
    case 1
        %BUCK mode
        if(Vin_in < uint32(5000))
            %Change to BOOST mode
            mode_out = uint8(2);
        end        
    case 2
        %BOOST mode
        %Change to DE_ENERGIZE mode
        mode_out = uint8(0);
    case 3
        %FAULT mode
        %Change to DE_ENERGIZE mode
        mode_out = uint8(3);
end

== matlab function BuckBoost/Vin_Vout ==
  data: Vin_i input; Vin_o output; Vout_i input; Vout_o output
function [Vin_o,Vout_o] = VinVoutCompute(Vin_i,Vout_i)
%#codegen
%VDDA = 3300

Vin_o = uint32(((Vin_i * 3300)/4095)*497/100);
Vout_o = uint32(((Vout_i * 3300)/4095)*503/100);

== matlab function BuckBoost/LedCompute ==
  data: Led3_out output; mode_in input; Vout_in input; Led5_out output; Led6_out output; mode_out output uint8
function [Led3_out,Led5_out,Led6_out,mode_out] = LedCompute(mode_in,Vout_in)
%#codegen
%Initialization
Led3_out = uint8(0);
Led5_out = uint8(0);
Led6_out = uint8(0);        
mode_out = mode_in;            
switch mode_in
    case 0
         %DE_ENERGISE mode
        if(Vout_in < uint32(2500))
            %Change to BUCK mode
            mode_out = uint8(1);            
        end 
        Led3_out = uint8(0);
        Led5_out = uint8(0);
        Led6_out = uint8(0);        
    case 1
        %BUCK mode
        Led3_out = uint8(0);
        Led5_out = uint8(1);
        Led6_out = uint8(0);                
    case 2
        %BOOST mode
        Led3_out = uint8(0);
        Led5_out = uint8(0);
        Led6_out = uint8(1);                        
    case 3
        %FAULT mode
        Led3_out = uint8(1);
        Led5_out = uint8(0);
        Led6_out = uint8(0);                        
end;
